simulink model "flux_linkage_ver1"  (R2020b)
settings: Solver=VariableStepAuto  StartTime=0.0  StopTime=1  RelTol=1e-3
InitFcn:
  | Rs=0.43;
  | 
  | Lls=0.002
  | 
  | Rr=0.816;
  | 
  | Llr=0.002
  | 
  | Lm=0.6931;
  | 
  | 
  | J=0.085;
  | np=2;
  | 
  | Ts=1e-5;
  | 
  | Udc=600*sqrt(3)
  | Tpwm = 4e-4;
  | 
  | Udc = 2700
  | J = 0.1
  | Llr = 0.006
  | Lls = 0.00116
  | Lm = 0.0254
  | Rr = 0.16
  | Rs = 0.15
  | 
  | Ls = 1.5*Lm+Lls
  | Lr = 1.5*Lm+Llr
  | Tr = Lr/Rr;
  | sigma = (Ls*Lr-Lm*Lm)/Ls/Lr;
model workspace (MAT data in the model file):
  Tsys = 2e-06
  sample_time = 1e-06
libraries: powerlib x10, simulink x2
settings Model: SimulationMode=accelerator  OrderedModelArguments=off  Creator=messer  LastModifiedBy=messer

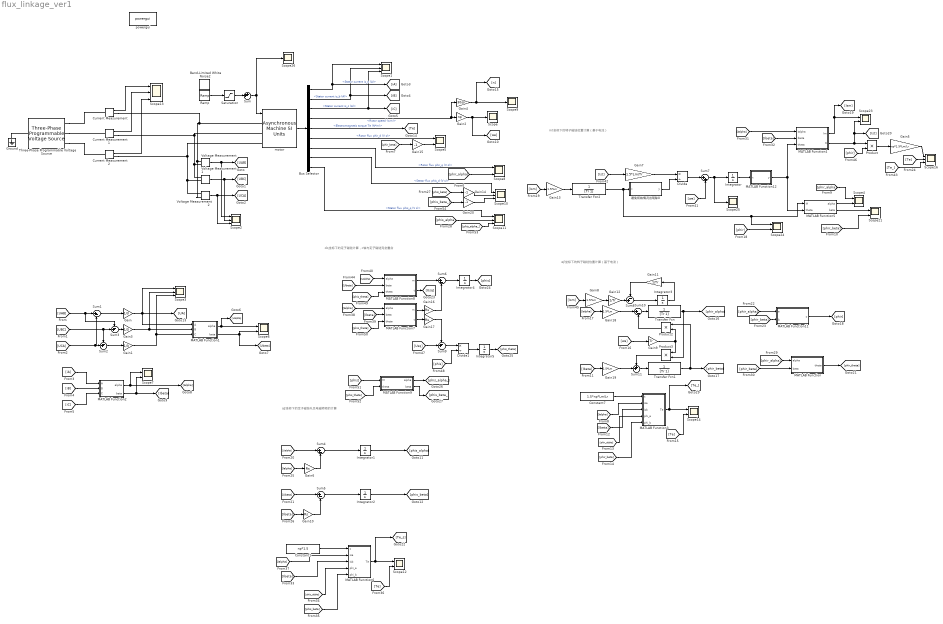
== system flux_linkage_ver1 ==
  note: αβ坐标下的转子磁链位置计算（基于电流）
  note: mt坐标下的转子磁链位置计算（基于电流）
  note: dq坐标下的定子磁链计算，d轴与定子磁链完全重合
  note: αβ坐标下的定子磁链以及电磁转矩的计算
  Band-Limited White Noise2 : simulink/Sources/Band-Limited White Noise  Cov=[0.0001]  Ts=1e-4  seed=[130341]
  Bus Selector : BusSelector  OutputSignals=Stator measurements.Stator current is_a (A),Stator measurements.Stator current is_b (A),Stator measurements.Stator current is_c (A),Mechanical.Rotor speed (wm),Mechanical.Electromagnetic torque Te (N*m),Rotor measurements.Rotor flux phir_d (V s),Rotor measurements.Rotor flux phir_q (V s),Stator measurements.Stator flux phis_d (V s),Stator measurements.Stator flux phis_q (V s)
  Constant1 : Constant  Value=np*1.5
  Constant7 : Constant  Value=1.5*np*Lm/Lr
  Current Measurement : powerlib/Measurements/Current Measurement  PhasorSimulation=off  OutputType=Complex  PSBequivalent=0
  Current Measurement1 : powerlib/Measurements/Current Measurement  PhasorSimulation=off  OutputType=Complex  PSBequivalent=0
  Current Measurement2 : powerlib/Measurements/Current Measurement  PhasorSimulation=off  OutputType=Complex  PSBequivalent=0
  Divide : Product  Inputs=*/
  Divide1 : Product  Inputs=*/
  Gain : Gain  Gain=1/3
  Gain1 : Gain  Gain=1/3
  Gain{6,10,16..17} (4 alike) : Gain  Gain=Rs
  Gain11 : Gain  Gain=1/Tr
  Gain12 : Gain  Gain=1/Tr
  Gain{8,13,18..19} (4 alike) : Gain  Gain=1.5*Lm
  Gain14 : Gain  Gain=-1
  Gain15 : Gain  Gain=-1
  Gain2 : Gain  Gain=np
  Gain20 : Gain  Gain=-1
  Gain3 : Gain  Gain=1/3
  Gain4 : Gain  Gain=30/pi
  Gain5 : Gain  Gain=np*1.5*Lm/Lr
  Gain7 : Gain  Gain=1.5*Lm/Tr
  Gain9 : Gain  Gain=Tr
  Ground : powerlib/Elements/Ground  LConnTagsString=a
  Integrator{,3..5} (4 alike) : Integrator  InitialCondition=1e-5
  Integrator1 : Integrator
  Integrator2 : Integrator
  MATLAB Function : MATLAB Function  TreatAsAtomicUnit=on
  MATLAB Function1 : MATLAB Function  TreatAsAtomicUnit=on
  MATLAB Function11 : MATLAB Function  TreatAsAtomicUnit=on
  MATLAB Function12 : MATLAB Function  TreatAsAtomicUnit=on
  MATLAB Function2 : MATLAB Function  TreatAsAtomicUnit=on
  MATLAB Function3 : MATLAB Function  TreatAsAtomicUnit=on
  MATLAB Function4 : MATLAB Function  TreatAsAtomicUnit=on
  MATLAB Function5 : MATLAB Function  TreatAsAtomicUnit=on
  MATLAB Function6 : MATLAB Function  TreatAsAtomicUnit=on
  MATLAB Function7 : MATLAB Function  TreatAsAtomicUnit=on
  MATLAB Function8 : MATLAB Function  TreatAsAtomicUnit=on
  MATLAB Function9 : MATLAB Function  TreatAsAtomicUnit=on
  Product : Product
  Product2 : Product
  Product3 : Product
  Ramp : simulink/Sources/Ramp  slope=100  start=0.15  InitialOutput=5
  Saturation : Saturate  UpperLimit=20  LowerLimit=0
  Scope{,9,25..26} (4 alike) : Scope
  Scope{1..3,10..11,13,16} (7 alike) : Scope  NumInputPorts=3
  Scope{4..8,12,14,21,23..24} (10 alike) : Scope  NumInputPorts=2
  Sum : Sum  Inputs=++|
  Sum{1,4..6,10} (5 alike) : Sum  Inputs=|+-
  Sum11 : Sum  Inputs=++|
  Sum{2..3,8..9} (4 alike) : Sum  Inputs=-+|
  Sum7 : Sum  Inputs=|++
  Three-Phase Programmable Voltage Source : powerlib/Electrical Sources/Three-Phase Programmable Voltage Source  PositiveSequence="[400*sqrt(2)  0 50]"  VariationEntity=None  VariationType=Table of time-amplitude pairs  VariationTypeAlt=Step  VariationStep=0.5  VariationRate=10  VariationMagnitude=0.3  VariationFrequency=2  VariationTiming=[1 2]  VariationPhaseA=off  Amplitudes=[1 0.8 1.2 1.0]  TimeValues=[0 0.1 0.15 0.2]  HarmonicGeneration=off  HarmonicA=[3 0.2 -25 0]  HarmonicB=[2 0.15 35 2]  Timing="[0.05  3]"  BusType=swing  Pref=0  Qref=0  Qmin=-inf  Qmax=inf
  Transfer Fcn : TransferFcn  Denominator=[Tr 1]
  Transfer Fcn1 : TransferFcn  Denominator=[Tr 1]
  Transfer Fcn2 : TransferFcn  Denominator=[Tr 1]
  Voltage Measurement : powerlib/Measurements/Voltage Measurement  PhasorSimulation=off  OutputType=Complex  PSBequivalent=0
  Voltage Measurement1 : powerlib/Measurements/Voltage Measurement  PhasorSimulation=off  OutputType=Complex  PSBequivalent=0
  Voltage Measurement2 : powerlib/Measurements/Voltage Measurement  PhasorSimulation=off  OutputType=Complex  PSBequivalent=0
  motor : powerlib/Machines/Asynchronous Machine SI Units  RotorType=Squirrel-cage  PresetModel=No  MechanicalLoad=Torque Tm  ShowDetailedParameters=on  ReferenceFrame=Stationary  Units=SI  MeasurementBus=off  NominalParameters=[562000 2750 135]  Stator=[Rs Lls]  Rotor=[Rr Llr]  Cage1=[0.4155 0.002066]  Cage2=[0.4168 0.0003495]  Lm=Lm  Mechanical=[J 0 np]  PolePairs=2  InitialConditions=[1 0 0 0 0 0 0 0]  SimulateSaturation=off  Saturation=[14.03593122, 27.81365428, 53.79336849, 72.68890987, 97.98006896, 148.6815601, 215.7428561, 302.9841135, 428.7778367 ; 230, 322, 414, 460, 506, 552, 598, 644, 690]  LoadFlowParameters=1492000  TsPowergui=0  TsBlock=-1  IterativeModel=Trapezoidal non iterative  IterativeDiscreteModel=Trapezoidal non iterative  Pmec=1.492e+006
  powergui : powerlib/powergui  Priority=1  SimulationMode=Discrete  SampleTime=Tsys  frequency=60  Iterations=50  frequencyindice=50  Pbase=100e6  ErrMax=1e-4  UnitsV=kV  UnitsW=MW  buscounter=0  FunctionMessages=off  echomessages=off  EnableUseOfTLC=off  CurrentSourceSwitches=off  DisableSnubberDevices=off  DisableRonSwitches=off  DisableVfSwitches=off  DisplayEquations=off  AutomaticDiscreteSolvers=off  SolverType=Tustin/Backward Euler (TBE)  Interpol=off  ExternalGateDelay=off  methode=off  Ts=100  x0status=blocks  SPID=on  SwTol=0  HookPort=off  NonlinearTolerance=1e-4  nMaxIteration=100  ContinueOnMaxIteration=off  RestoreLinks=warning  ResistiveCurrentMeasurement=off  Frange=[0:2:500]  Ylog=off  Xlog=on  ShowGrid=off  save=off  variable=ZData  structure=0  ZoomFFT=off  StartTime=0.0  cycles=1  DisplayStyle=1  fundamental=60  FreqAxis=off  MaxFrequency=1000  frequencyindicesteady=1  RmsSteady=1  display=off
  避免初始情况出现除0 : MATLAB Function  TreatAsAtomicUnit=on
  wires:
  Bus Selector/4 -> Gain4/1, Gain2/1  "<Rotor speed (wm)>"
  Bus Selector/2 -> [iB], Scope1/2  "<Stator current is_b (A)>"
  Bus Selector/5 -> [Te]  "<Electromagnetic torque Te (N*m)>"
  Saturation/1 -> Sum/2
  Bus Selector/1 -> [iA], Scope1/1  "<Stator current is_a (A)>"
  motor/1 -> Bus Selector/1
  Bus Selector/3 -> [iC], Scope1/3  "<Stator current is_c (A)>"
  Ramp/1 -> Saturation/1
  Voltage Measurement1/1 -> [UBC], Scope2/2
  Voltage Measurement/1 -> Scope2/1, [UAB]
  Voltage Measurement2/1 -> [UCA], Scope2/3
  [UAB] -> Sum3/1, Sum1/1
  [UCA] -> Sum1/2, Sum2/2
  Sum1/1 -> Gain/1
  [UBC] -> Sum2/1, Sum3/2
  Sum2/1 -> Gain1/1
  Sum3/1 -> Gain3/1
  Gain3/1 -> MATLAB Function1/2(B), Scope3/2
  Gain/1 -> MATLAB Function1/1(A), [UA], Scope3/1
  Gain1/1 -> MATLAB Function1/3(C), Scope3/3
  Sum/1 -> Scope26/1, motor/1
  MATLAB Function1/1(alpha) -> [Ualpha], Scope6/1
  MATLAB Function1/2(beta) -> [Ubeta], Scope6/2
  MATLAB Function2/2(beta) -> [Ibeta], Scope7/2
  [iB] -> MATLAB Function2/2(B)
  MATLAB Function2/1(alpha) -> Scope7/1, [Ialpha]
  [phir_alpha] -> Scope8/2
  [phir_beta] -> Gain15/1
  Gain15/1 -> Scope5/2
  Bus Selector/6 -> Scope5/1  "<Rotor flux phir_d (V s)>"
  Bus Selector/7 -> Scope8/1  "<Rotor flux phir_q (V s)>"
  Gain2/1 -> [we], Scope/1
  [iA] -> MATLAB Function2/1(A)
  [iC] -> MATLAB Function2/3(C)
  Constant7/1 -> MATLAB Function3/1(c)
  [Ialpha] -> MATLAB Function3/2(isa)
  [Ibeta] -> MATLAB Function3/3(isb)
  [phir_alpha] -> MATLAB Function3/4(phi_a)
  [phir_beta] -> MATLAB Function3/5(phi_b)
  MATLAB Function3/1(Te) -> [Te_], Scope14/1
  [Te] -> Scope14/2
  Gain4/1 -> [n], Scope9/1
  Current Measurement1/1 -> Scope13/2
  Current Measurement2/1 -> Scope13/3
  Current Measurement/1 -> Scope13/1
  [Ialpha] -> MATLAB Function4/1(Ialpha)
  [Ibeta] -> MATLAB Function4/2(Ibeta)
  MATLAB Function4/2(It) -> Scope23/2, [Ist], Product/1
  Product/1 -> Gain5/1
  Gain5/1 -> Scope16/1
  [Te] -> Scope16/2
  MATLAB Function4/1(Im) -> [Ism], Scope23/1
  [Ist] -> Gain7/1
  Gain7/1 -> Divide/1
  Divide/1 -> Sum7/1
  [we] -> Sum7/2
  Sum7/1 -> Scope25/1, Integrator/1
  [Ism] -> Gain8/1
  [phir] -> Product/2
  Gain8/1 -> Gain12/1
  Integrator3/1 -> Gain11/1
  Sum8/1 -> Integrator3/1
  Integrator/1 -> MATLAB Function12/1(x)
  Gain11/1 -> Sum8/1
  Gain12/1 -> Sum8/2
  Sum10/1 -> Transfer Fcn/1
  Gain18/1 -> Sum10/1
  Sum11/1 -> Transfer Fcn1/1
  Product2/1 -> Sum10/2
  Gain19/1 -> Sum11/2
  [Ibeta] -> Gain19/1
  [Ialpha] -> Gain18/1
  Transfer Fcn/1 -> Product3/2, [phir_alpha]
  [we] -> Gain9/1
  Product3/1 -> Sum11/1
  Gain9/1 -> Product3/1, Product2/2
  Transfer Fcn1/1 -> Product2/1, [phir_beta]
  [phir_alpha] -> MATLAB Function11/1(a)
  [phir_beta] -> MATLAB Function11/2(b)
  [phir_beta] -> MATLAB Function/2(beta)
  [phir_alpha] -> MATLAB Function/1(alpha)
  MATLAB Function11/1(y) -> [phir]
  MATLAB Function/1(theta) -> [phir_theta]
  MATLAB Function12/1(y) -> MATLAB Function4/3(theta), MATLAB Function5/2(theta)
  MATLAB Function5/1(alpha) -> Scope4/2
  [phir_alpha] -> Scope4/1
  MATLAB Function5/2(beta) -> Scope21/1
  [phir_beta] -> Scope21/2
  [phir] -> Scope24/2
  [Ism] -> Gain13/1
  Gain13/1 -> Transfer Fcn2/1
  避免初始情况出现除0/1(y) -> Divide/2
  Transfer Fcn2/1 -> Scope24/1, MATLAB Function5/1(M), 避免初始情况出现除0/1(x)
  [Te_] -> Scope16/3
  [Ualpha] -> Sum4/1
  [Ialpha] -> Gain6/1
  Gain6/1 -> Sum4/2
  Sum4/1 -> Integrator1/1
  [Ubeta] -> Sum5/1
  [Ibeta] -> Gain10/1
  Gain10/1 -> Sum5/2
  Sum5/1 -> Integrator2/1
  Integrator1/1 -> [phis_alpha]
  Integrator2/1 -> [phis_beta]
  Gain14/1 -> Scope10/2
  [phis_beta] -> Gain14/1
  Bus Selector/8 -> Scope10/1  "<Stator flux phis_d (V s)>"
  [phis_alpha] -> Scope11/2
  Bus Selector/9 -> Scope11/1  "<Stator flux phis_q (V s)>"
  [Te] -> Scope12/2
  MATLAB Function6/1(Te) -> Scope12/1, [Te_s]
  [phis_beta] -> MATLAB Function6/5(phi_b)
  [phis_alpha] -> MATLAB Function6/4(phi_a)
  [Ibeta] -> MATLAB Function6/3(isb)
  [Ialpha] -> MATLAB Function6/2(isa)
  Constant1/1 -> MATLAB Function6/1(c)
  [Ibeta] -> MATLAB Function7/2(beta)
  [Ialpha] -> MATLAB Function7/1(alpha)
  [Ualpha] -> MATLAB Function8/1(alpha)
  [Ubeta] -> MATLAB Function8/2(beta)
  MATLAB Function7/1(m) -> Gain16/1
  MATLAB Function8/1(m) -> Sum6/1
  Gain16/1 -> Sum6/2
  Sum6/1 -> Integrator4/1
  MATLAB Function8/2(t) -> [Usq]
  [Usq] -> Sum9/2
  MATLAB Function7/2(t) -> Gain17/1
  Gain17/1 -> Sum9/1
  Integrator4/1 -> [phis]
  Sum9/1 -> Divide1/1
  [phis] -> Divide1/2
  Divide1/1 -> Integrator5/1
  Integrator5/1 -> [phis_theta]
  [phis_theta] -> MATLAB Function8/3(theta)
  [phis_theta] -> MATLAB Function7/3(theta)
  [phis] -> MATLAB Function9/1(M)
  [phis_theta] -> MATLAB Function9/2(theta)
  MATLAB Function9/1(alpha) -> [phis_alpha_]
  MATLAB Function9/2(beta) -> [phis_beta_]
  [phis_beta_] -> Gain20/1
  Gain20/1 -> Scope10/3
  [phis_alpha_] -> Scope11/3
  connections:
  Voltage Measurement1/LConn1 -- Voltage Measurement/LConn2 -- motor/LConn2 -- Current Measurement1/RConn1
  Voltage Measurement2/LConn1 -- Voltage Measurement1/LConn2 -- Current Measurement2/RConn1 -- motor/LConn3
  Voltage Measurement/LConn1 -- Voltage Measurement2/LConn2 -- Current Measurement/RConn1 -- motor/LConn1
  Ground/LConn1 -- Three-Phase Programmable Voltage Source/LConn1
  Three-Phase Programmable Voltage Source/RConn2 -- Current Measurement1/LConn1
  Three-Phase Programmable Voltage Source/RConn1 -- Current Measurement/LConn1
  Three-Phase Programmable Voltage Source/RConn3 -- Current Measurement2/LConn1

== matlab function flux_linkage_ver1/MATLAB Function9 ==
  data: alpha output; M input; theta input; beta output
function [alpha, beta] = fcn(M, theta)

alpha = M * cos(theta);
beta = M * sin(theta);

== matlab function flux_linkage_ver1/MATLAB Function ==
  data: theta output; alpha input; beta input
function theta = fcn(alpha, beta)

if(beta >=0)
    if(alpha == 0)
        theta = pi/2;
    elseif(alpha >0)
        theta = atan(beta/alpha);
    else
        theta = pi + atan(beta/alpha);
    end
else
    if(alpha == 0)
        theta = 1.5*pi;
    elseif(alpha > 0)
        theta = 2*pi + atan(beta/alpha);
    else
        theta = pi + atan(beta/alpha);
    end
end

== matlab function flux_linkage_ver1/MATLAB Function1 ==
  data: A input; alpha output; B input; C input; beta output
function [alpha, beta] = fcn(A, B, C)
k = 2/ 3;
alpha = k * (A - 0.5*B - 0.5*C);
beta = k * sqrt(3) / 2 * (B - C);

== matlab function flux_linkage_ver1/MATLAB Function12 ==
  data: y output; x input
function y = fcn(x)

y = mod(x, 2*pi);

== matlab function flux_linkage_ver1/避免初始情况出现除0 ==
  data: y output; x input
function y = fcn(x)

if(x==0)
    y = 1;
else
    y = x;
end

== matlab function flux_linkage_ver1/MATLAB Function5 ==
  data: alpha output; M input; theta input; beta output
function [alpha, beta] = fcn(M, theta)

alpha = M * cos(theta);
beta = M * sin(theta);

== matlab function flux_linkage_ver1/MATLAB Function2 ==
  data: A input; alpha output; B input; C input; beta output
function [alpha, beta] = fcn(A, B, C)
k = 2/ 3;
alpha = k * (A - 0.5*B - 0.5*C);
beta = k * sqrt(3) / 2 * (B - C);

== matlab function flux_linkage_ver1/MATLAB Function3 ==
  data: c input; Te output; isa input; isb input; phi_a input; phi_b input
function Te = fcn(c, isa, isb, phi_a, phi_b)
Te = c *( isb * phi_a - isa * phi_b);

== matlab function flux_linkage_ver1/MATLAB Function4 ==
  data: Im output; Ialpha input; Ibeta input; theta input; It output
function [Im, It] = fcn(Ialpha, Ibeta, theta)

Im = Ialpha * cos(theta) + Ibeta * sin(theta);
It = -Ialpha * sin(theta) + Ibeta * cos(theta);

== matlab function flux_linkage_ver1/MATLAB Function11 ==
  data: y output; a input; b input
function y = fcn(a, b)

y = sqrt(a*a + b*b);

== matlab function flux_linkage_ver1/MATLAB Function6 ==
  data: c input; Te output; isa input; isb input; phi_a input; phi_b input
function Te = fcn(c, isa, isb, phi_a, phi_b)
Te = c *( isb * phi_a - isa * phi_b);

== matlab function flux_linkage_ver1/MATLAB Function7 ==
  data: m output; alpha input; beta input; theta input; t output
function [m, t] = fcn(alpha, beta, theta)

m = alpha * cos(theta) + beta * sin(theta);
t = -alpha * sin(theta) + beta * cos(theta);

== matlab function flux_linkage_ver1/MATLAB Function8 ==
  data: m output; alpha input; beta input; theta input; t output
function [m, t] = fcn(alpha, beta, theta)

m = alpha * cos(theta) + beta * sin(theta);
t = -alpha * sin(theta) + beta * cos(theta);
